simulink model "chap8_1sim"  (Simulink 6.3)
settings: Solver=ode45  StartTime=0.0  StopTime=30  RelTol=1e-5
settings Model: Creator=hp  LastModifiedBy=Administrator  ExtModeTrigMode=oneshot  ExtModeArmWhenConnect=off
settings DataIOCC: LimitDataPoints=off  SignalLoggingName=sigsOut
settings OptimizationCC: BooleanDataType=off
settings DebuggingCC: SolverPrmCheckMsg=none
settings HardwareCC: TargetUnknown=on

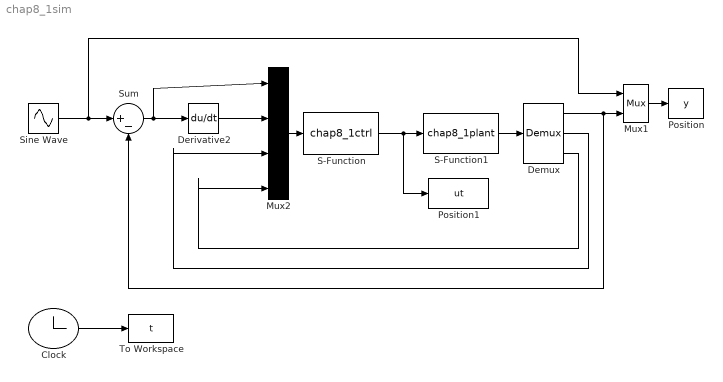
== system chap8_1sim ==
  Clock : Clock
      settings: Decimation=10
  Demux : Demux  Outputs=3
  Derivative2 : Derivative
  Mux1 : Mux  Inputs=2
  Mux2 : Mux
  Position : ToWorkspace  VariableName=y  SampleTime=-1  SaveFormat=Array
  Position1 : ToWorkspace  VariableName=ut  SampleTime=-1  SaveFormat=Array
  S-Function : S-Function  FunctionName=chap8_1ctrl
  S-Function1 : S-Function  FunctionName=chap8_1plant
  Sine Wave : Sin  Amplitude=0.1  SampleTime=0
  Sum : Sum  Inputs=|+-  SaturateOnIntegerOverflow=on
  To Workspace : ToWorkspace  VariableName=t  SampleTime=-1  SaveFormat=Array
  wires:
  Mux1/1 -> Position/1
  S-Function1/1 -> Demux/1
  S-Function/1 -> S-Function1/1, Position1/1
  Clock/1 -> To Workspace/1
  Sine Wave/1 -> Sum/1, Mux1/1
  Mux2/1 -> S-Function/1
  Sum/1 -> Mux2/1, Derivative2/1
  Derivative2/1 -> Mux2/2
  Demux/2 -> Mux2/3
  Demux/3 -> Mux2/4
  Demux/1 -> Mux1/2, Sum/2
